simulink model "title1"  (R2019a)
settings: Solver=VariableStepAuto  StartTime=0.0  StopTime=30.0  RelTol=1e-3
settings Model: Creator=慈凌宇  LastModifiedBy=慈凌宇

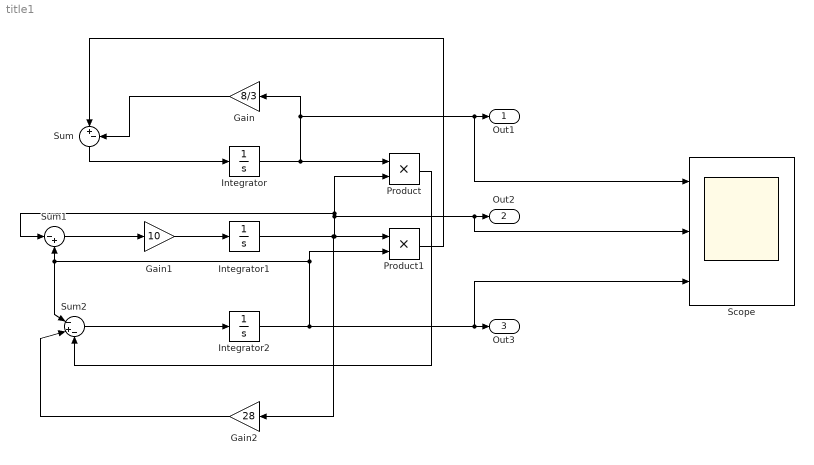
== system title1 ==
  Gain : Gain  Gain=8/3
  Gain1 : Gain  Gain=10
  Gain2 : Gain  Gain=28
  Integrator : Integrator
  Integrator1 : Integrator
  Integrator2 : Integrator  InitialCondition=1e-3
  Product : Product
  Product1 : Product
  Scope : Scope  NumInputPorts=3
  Sum : Sum  Inputs=|+-
  Sum1 : Sum  Inputs=|-+
  Sum2 : Sum  Inputs=|-+-
  Out1 : Outport  SignalName=out1
  Out2 : Outport  Port=2  SignalName=out2
  Out3 : Outport  Port=3  SignalName=out3
  wires:
  Integrator/1 -> Scope/1, Out1/1, Gain/1, Product/1
  Gain/1 -> Sum/2
  Integrator1/1 -> Gain2/1, Product1/1, Sum1/1, Product/2, Scope/2, Out2/1
  Gain1/1 -> Integrator1/1
  Sum/1 -> Integrator/1
  Product1/1 -> Sum/1
  Sum1/1 -> Gain1/1
  Integrator2/1 -> Scope/3, Out3/1, Sum2/1, Sum1/2, Product1/2
  Gain2/1 -> Sum2/2
  Product/1 -> Sum2/3
  Sum2/1 -> Integrator2/1
